simulink model "model_2022b1"  (R2023b)
settings: Solver=FixedStepAuto  StartTime=0.0  StopTime=Tmdl  FixedStep=0.001  RelTol=1e-3
undefined symbols (not defined in the file): A, A0g, AM, b, b0g, C, gamma, K
settings Model: Creator=Катя  LastModifiedBy=deniskirbaba

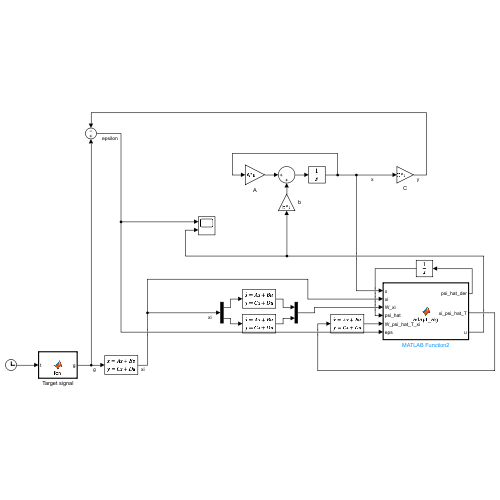
[thumbnail: Simulink's stored preview of the top-level diagram]
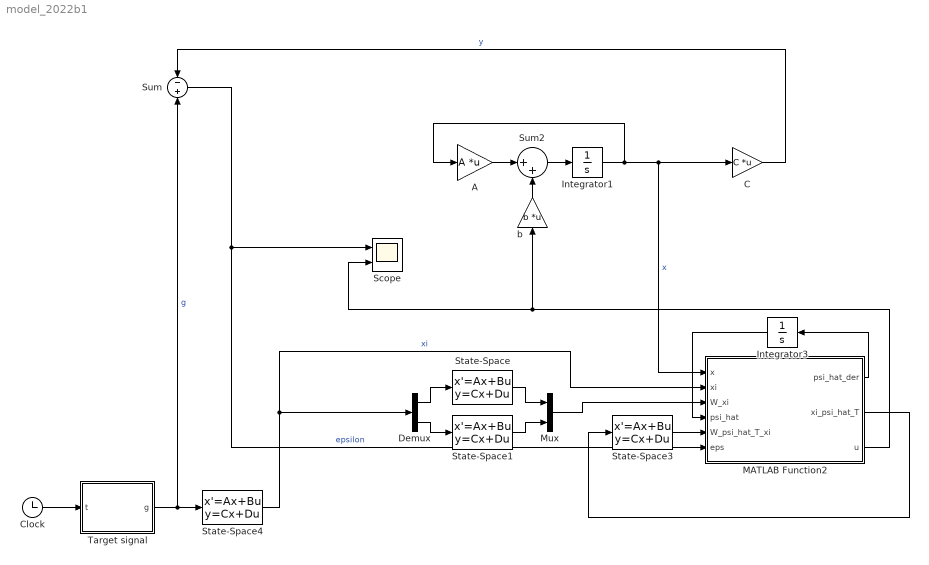
== system model_2022b1 ==
  A : Gain  Gain=A  Multiplication=Matrix(K*u)
  C : Gain  Gain=C  Multiplication=Matrix(K*u)
  Clock : Clock
  Demux : Demux  Outputs=2
  Integrator1 : Integrator  InitialCondition=[0;0]
  Integrator3 : Integrator  InitialCondition=[0;0]
  MATLAB Function2 : MATLAB Function  TreatAsAtomicUnit=on
  Mux : Mux  Inputs=2
  Scope : Scope  NumInputPorts=2
  State-Space : StateSpace  A=AM  B=b  C=C  D=0  InitialCondition=0
  State-Space1 : StateSpace  A=AM  B=b  C=C  D=0  InitialCondition=0
  State-Space3 : StateSpace  A=AM  B=b  C=C  D=0  InitialCondition=0
  State-Space4 : StateSpace  A=A0g  B=b0g  C=eye(2)  D=[0;0]  InitialCondition=0  ParameterTunability=Unconstrained
  Sum : Sum  Inputs=-+
  Sum2 : Sum  Inputs=|++
  Target signal : MATLAB Function  TreatAsAtomicUnit=on
  b : Gain  Gain=b  Multiplication=Matrix(K*u)
  wires:
  Integrator1/1 -> MATLAB Function2/1(x), C/1, A/1  "x"
  MATLAB Function2/1(psi_hat_der) -> Integrator3/1
  A/1 -> Sum2/1
  b/1 -> Sum2/2
  Sum2/1 -> Integrator1/1
  Target signal/1(g) -> State-Space4/1, Sum/2  "g"
  Clock/1 -> Target signal/1(t)
  C/1 -> Sum/1  "y"
  Mux/1 -> MATLAB Function2/3(W_xi)
  State-Space/1 -> Mux/1
  Demux/1 -> State-Space/1
  State-Space1/1 -> Mux/2
  Demux/2 -> State-Space1/1
  State-Space3/1 -> MATLAB Function2/5(W_psi_hat_T_xi)
  State-Space4/1 -> MATLAB Function2/2(xi), Demux/1  "xi"
  Integrator3/1 -> MATLAB Function2/4(psi_hat)
  MATLAB Function2/3(u) -> Scope/2, b/1
  Sum/1 -> MATLAB Function2/6(eps), Scope/1  "epsilon"
  MATLAB Function2/2(xi_psi_hat_T) -> State-Space3/1

== matlab function model_2022b1/MATLAB Function2 ==
  data: x input; xi input; W_xi input; psi_hat input; W_psi_hat_T_xi input; psi_hat_der output; gamma parameter; eps input; xi_psi_hat_T output; u output; K parameter
function [psi_hat_der, xi_psi_hat_T,u]  = adapt_alg(x,xi,W_xi, psi_hat, W_psi_hat_T_xi, gamma, eps, K)

    xi_psi_hat_T = xi'*psi_hat;
    eps_hat = eps - psi_hat'*W_xi + W_psi_hat_T_xi;
    u = -K*x + psi_hat'*xi;
    psi_hat_der = gamma*W_xi*eps_hat;
    
end

== matlab function model_2022b1/Target signal ==
  data: t input; g output
function g = fcn(t)

g = 5*cos(5*t+1.5);
